simulink model "flattening_2_test"  (Simulink 7.2)
settings: Solver=VariableStepDiscrete  StartTime=0.0  StopTime=10.0  RelTol=1e-3
settings Model: Creator=arnaud  LastModifiedBy=arnaud

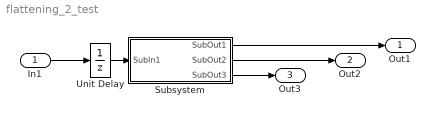
== system flattening_2_test ==
  In1 : Inport  OutDataType=sfix(16)  OutScaling=2^0
  Subsystem : Subsystem
  Unit Delay : UnitDelay
  Out1 : Outport  OutDataType=sfix(16)  OutScaling=2^0
  Out2 : Outport  Port=2  OutDataType=sfix(16)  OutScaling=2^0
  Out3 : Outport  Port=3  OutDataType=sfix(16)  OutScaling=2^0
  wires:
  Subsystem/1(SubOut1) -> Out1/1
  Subsystem/2(SubOut2) -> Out2/1
  Unit Delay/1 -> Subsystem/1(SubIn1)
  In1/1 -> Unit Delay/1
  Subsystem/3(SubOut3) -> Out3/1

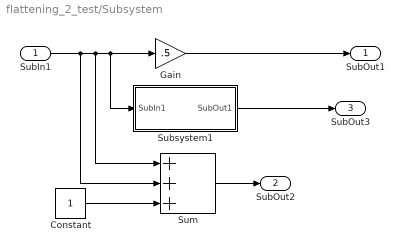
== system flattening_2_test/Subsystem ==
  SubIn1 : Inport  OutDataType=sfix(16)  OutScaling=2^0
  Constant : Constant  OutDataType=sfix(16)  OutScaling=2^0
  Gain : Gain  Gain=.5  ParameterDataType=sfix(16)  ParameterScaling=2^0  OutDataType=sfix(16)  OutScaling=2^0
  Subsystem1 : Subsystem
  Sum : Sum  Inputs=+++  OutDataType=sfix(16)  OutScaling=2^0
  SubOut1 : Outport  OutDataType=sfix(16)  OutScaling=2^0
  SubOut2 : Outport  Port=2  OutDataType=sfix(16)  OutScaling=2^0
  SubOut3 : Outport  Port=3  OutDataType=sfix(16)  OutScaling=2^0
  wires:
  SubIn1/1 -> Subsystem1/1(SubIn1), Gain/1, Sum/1, Sum/2
  Gain/1 -> SubOut1/1
  Sum/1 -> SubOut2/1
  Constant/1 -> Sum/3
  Subsystem1/1(SubOut1) -> SubOut3/1

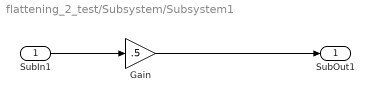
== system flattening_2_test/Subsystem/Subsystem1 ==
  SubIn1 : Inport  OutDataType=sfix(16)  OutScaling=2^0
  Gain : Gain  Gain=.5  ParameterDataType=sfix(16)  ParameterScaling=2^0  OutDataType=sfix(16)  OutScaling=2^0
  SubOut1 : Outport  OutDataType=sfix(16)  OutScaling=2^0
  wires:
  Gain/1 -> SubOut1/1
  SubIn1/1 -> Gain/1
